simulink model "while_ex"  (R2018a)
settings: Solver=VariableStepAuto  StartTime=0.0  StopTime=10.0  RelTol=1e-3
settings Model: Creator=lenovo  LastModifiedBy=DELL

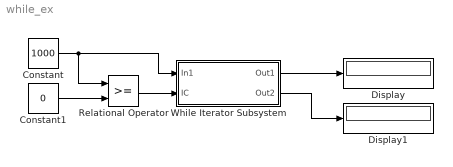
== system while_ex ==
  Constant : Constant  Value=1000
  Constant1 : Constant  Value=0
  Display : Display
  Display1 : Display
  Relational Operator : RelationalOperator  OutDataTypeStr=boolean  RndMeth=Simplest
  While Iterator Subsystem : Subsystem  TreatAsAtomicUnit=on
  wires:
  Constant/1 -> Relational Operator/1, While Iterator Subsystem/1(In1)
  Constant1/1 -> Relational Operator/2
  While Iterator Subsystem/1(Out1) -> Display/1
  Relational Operator/1 -> While Iterator Subsystem/2(IC)
  While Iterator Subsystem/2(Out2) -> Display1/1

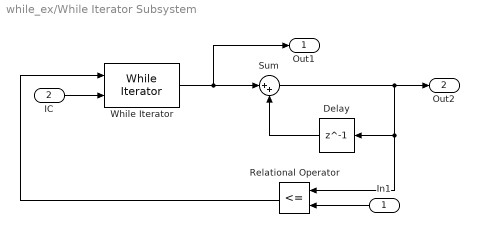
== system while_ex/While Iterator Subsystem ==
  In1 : Inport
  IC : Inport  Port=2
  Delay : Delay  DelayLength=1  InitialCondition=0
  Relational Operator : RelationalOperator  Operator=<=  OutDataTypeStr=boolean  RndMeth=Simplest
  Sum : Sum  Inputs=|++
  While Iterator : WhileIterator  MaxIters=100  ResetStates=reset  ShowIterationPort=on  OutputDataType=double
  Out1 : Outport  VectorParamsAs1DForOutWhenUnconnected=off
  Out2 : Outport  Port=2  VectorParamsAs1DForOutWhenUnconnected=off
  wires:
  IC/1 -> While Iterator/2
  In1/1 -> Relational Operator/2
  Delay/1 -> Sum/2
  Sum/1 -> Out2/1, Relational Operator/1, Delay/1
  While Iterator/1 -> Out1/1, Sum/1
  Relational Operator/1 -> While Iterator/1
